simulink model "crazyflie"  (R2019a)
settings: Solver=FixedStepDiscrete  StartTime=0.0  StopTime=25  FixedStep=0.01  RelTol=1e-3
values from neighbouring files (symbols this model uses):
  g = 9.81    [linearization.m]    (also in main.m)
  H = zeros(3,length(idx));  H(1,1) = 1; H(2,2) = 1; H(3,5) = 1    [main.m]
  K_fb_int = K    [main.m]
  K_fb_ref = K    [main.m]
  Kr = pinv( H * inv(eye(size(Ar)) + Br*K_fb_ref - Ar) * Br )    [main.m]
  x0 = [0 0 0  0 0 0  deg2rad(20) deg2rad(20) deg2rad(0) 0 0 0]'    [main.m]
undefined symbols (not defined in the file or in its folder): DiscIntNeverNeededParam
libraries: simulink x2, simulink_extras x1
settings Model: PauseTimes=7  Creator=Zrean  LastModifiedBy=lucas
settings DataIOCC: ReturnWorkspaceOutputs=off
settings OptimizationCC: DefaultParameterBehavior=Inlined  UseDivisionForNetSlopeComputation=on  UseFloatMulNetSlope=on  UseSpecifiedMinMax=on  InlineInvariantSignals=on  PassReuseOutputArgsAs=Individual arguments  ZeroExternalMemoryAtStartup=off  ZeroInternalMemoryAtStartup=off  NoFixptDivByZeroProtection=on  EfficientFloat2IntCast=on  LifeSpan=1
settings DebuggingCC: AlgebraicLoopMsg=error  ParameterTunabilityLossMsg=error  ArithmeticOperatorsInVariantConditions=warning
settings HardwareCC: ProdBitPerPointer=32  ProdBitPerSizeT=32  ProdBitPerPtrDiffT=32  ProdLargestAtomicInteger=Long  ProdLargestAtomicFloat=Double  ProdWordSize=32  ProdHWDeviceType=ARM Compatible->ARM Cortex
settings SFSimCC: SimUseLocalCustomCode=off  MATLABDynamicMemAlloc=off
settings RTWCC: SystemTargetFile=ert.tlc  GenCodeOnly=on  TemplateMakefile=ert_default_tmf  GenerateReport=on  RTWUseLocalCustomCode=off  BuildConfiguration=Faster Runs  IncludeHyperlinkInReport=on  LaunchReport=on  GenerateTraceInfo=on  GenerateTraceReport=on  GenerateTraceReportSl=on  GenerateTraceReportSf=on  GenerateTraceReportEml=on  GenerateCodeMetricsReport=on
settings CodeAppCC: ForceParamTrailComments=on  IgnoreCustomStorageClasses=off  OperatorAnnotations=on  SimulinkDataObjDesc=on  SFDataObjDesc=on  MATLABFcnDesc=on  CustomSymbolStrGlobalVar=rt$N$M  CustomSymbolStrType=$N$M  CustomSymbolStrFcn=$N$M$F  CustomSymbolStrMacro=$N$M  InsertBlockDesc=on  StateflowObjectComments=on  MATLABSourceComments=on
settings ERTTargetCC: TargetLangStandard=C99 (ISO)  MultiwordLength=2048  CombineSignalStateStructs=on  SuppressErrorStatus=on  SupportNonFinite=off  SupportComplex=off  InlinedParameterPlacement=NonHierarchical  ERTCustomFileTemplate=crazyflie_wrapper.tlc  ERTFilePackagingFormat=CompactWithDataFile
settings SimscapeCC: SimscapeNormalizeSystem=off

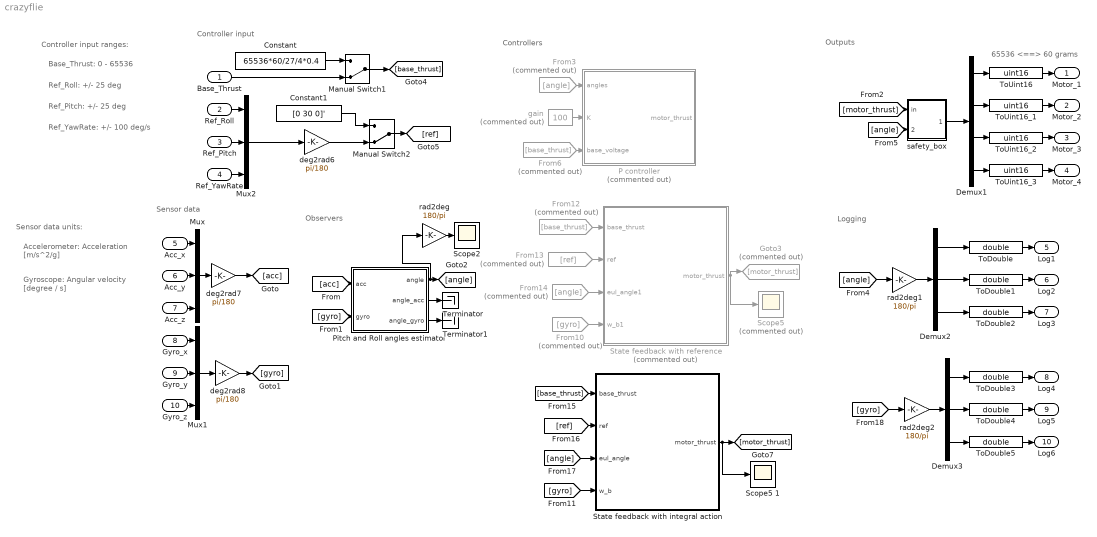
== system crazyflie ==
  note: 65536 <==> 60 grams
  note: Ref_Roll: +/- 25 deg
  note: Base_Thrust: 0 - 65536
  note: Ref_Pitch: +/- 25 deg
  note: Ref_YawRate: +/- 100 deg/s
  note: Controller input ranges:
  note: Gyroscope:
      | Angular velocity [degree / s]
  note: Accelerometer:
      | Acceleration [m/s^2/g]
  note: Sensor data units:
  note: Logging
  note: Outputs
  note: Sensor data
  note: Controllers
  note: Controller input
  note: Observers
  Base_Thrust : Inport  OutDataTypeStr=double
  Ref_Roll : Inport  Port=2  OutDataTypeStr=double
  Ref_Pitch : Inport  Port=3  OutDataTypeStr=double
  Ref_YawRate : Inport  Port=4  OutDataTypeStr=double
  Acc_x : Inport  Port=5  OutDataTypeStr=double  PortDimensions=1
  Acc_y : Inport  Port=6  OutDataTypeStr=double  PortDimensions=1
  Acc_z : Inport  Port=7  OutDataTypeStr=double  PortDimensions=1
  Gyro_x : Inport  Port=8  OutDataTypeStr=double  PortDimensions=1
  Gyro_y : Inport  Port=9  OutDataTypeStr=double  PortDimensions=1
  Gyro_z : Inport  Port=10  OutDataTypeStr=double  PortDimensions=1
  Constant : Constant  Value=65536*60/27/4*0.4
  Constant1 : Constant  Value=[0 30 0]'
  Demux1 : Demux
  Demux2 : Demux  Outputs=3
  Demux3 : Demux  Outputs=3
  From10 : From  Commented=on  GotoTag=gyro
  From12 : From  Commented=on  GotoTag=base_thrust
  From13 : From  Commented=on  GotoTag=ref
  From14 : From  Commented=on  GotoTag=angle
  From3 : From  Commented=on  GotoTag=angle
  From6 : From  Commented=on  GotoTag=base_thrust
  Goto3 : Goto  Commented=on  GotoTag=motor_thrust
  Manual Switch1 : ManualSwitch  CurrentSetting=0
  Manual Switch2 : ManualSwitch  CurrentSetting=0
  Mux : Mux  Inputs=3
  Mux1 : Mux  Inputs=3
  Mux2 : Mux  Inputs=3
  P controller : MATLAB Function  Commented=on  TreatAsAtomicUnit=on
  Pitch and Roll angles estimator : Subsystem
  Scope2 : Scope
  "Scope5 " : Scope  Commented=on
  Scope5 1 : Scope
  State feedback with integral action : Subsystem
  State feedback with reference : Subsystem  Commented=on
  Terminator : Terminator
  Terminator1 : Terminator
  ToDouble{,1..5} (6 alike) : DataTypeConversion  OutDataTypeStr=double  SaturateOnIntegerOverflow=on
  ToUint16 : DataTypeConversion  OutDataTypeStr=uint16  SaturateOnIntegerOverflow=on
  ToUint16_1 : DataTypeConversion  OutDataTypeStr=uint16  SaturateOnIntegerOverflow=on
  ToUint16_2 : DataTypeConversion  OutDataTypeStr=uint16  SaturateOnIntegerOverflow=on
  ToUint16_3 : DataTypeConversion  OutDataTypeStr=uint16  SaturateOnIntegerOverflow=on
  deg2rad6 : Gain  Gain=pi/180
  deg2rad7 : Gain  Gain=pi/180
  deg2rad8 : Gain  Gain=pi/180
  gain : Constant  Commented=on  Value=100
  rad2deg : Gain  Gain=180/pi
  rad2deg1 : Gain  Gain=180/pi
  rad2deg2 : Gain  Gain=180/pi
  safety_box : Subsystem
  Motor_1 : Outport  OutDataTypeStr=uint16  LockScale=on
  Motor_2 : Outport  Port=2  OutDataTypeStr=uint16  LockScale=on
  Motor_3 : Outport  Port=3  OutDataTypeStr=uint16  LockScale=on
  Motor_4 : Outport  Port=4  OutDataTypeStr=uint16  LockScale=on
  Log1 : Outport  Port=5  OutDataTypeStr=double
  Log2 : Outport  Port=6  OutDataTypeStr=double
  Log3 : Outport  Port=7  OutDataTypeStr=double
  Log4 : Outport  Port=8  OutDataTypeStr=double
  Log5 : Outport  Port=9  OutDataTypeStr=double
  Log6 : Outport  Port=10  OutDataTypeStr=double
  wires:
  ToUint16/1 -> Motor_1/1
  ToUint16_1/1 -> Motor_2/1
  ToUint16_2/1 -> Motor_3/1
  ToUint16_3/1 -> Motor_4/1
  ToDouble/1 -> Log1/1
  ToDouble1/1 -> Log2/1
  ToDouble2/1 -> Log3/1
  ToDouble3/1 -> Log4/1
  ToDouble4/1 -> Log5/1
  ToDouble5/1 -> Log6/1
  State feedback with reference/1(motor_thrust) -> Goto3/1, "Scope5 "/1
  [ref] -> State feedback with integral action/2(ref)
  Demux2/3 -> ToDouble2/1
  From12/1 -> State feedback with reference/1(base_thrust)
  [acc] -> Pitch and Roll angles estimator/1(acc)
  State feedback with integral action/1(motor_thrust) -> Scope5 1/1, [motor_thrust]
  Pitch and Roll angles estimator/2(angle_acc) -> Terminator/1
  From6/1 -> P controller/3(base_voltage)
  Pitch and Roll angles estimator/3(angle_gyro) -> Terminator1/1
  Demux2/2 -> ToDouble1/1
  [gyro] -> State feedback with integral action/4(w_b)
  [angle] -> rad2deg1/1
  From3/1 -> P controller/1(angles)
  gain/1 -> P controller/2(K)
  [angle] -> State feedback with integral action/3(eul_angle)
  Pitch and Roll angles estimator/1(angle) -> rad2deg/1, [angle]
  Demux2/1 -> ToDouble/1
  [gyro] -> Pitch and Roll angles estimator/2(gyro)
  [base_thrust] -> State feedback with integral action/1(base_thrust)
  From14/1 -> State feedback with reference/3(eul_angle1)
  From10/1 -> State feedback with reference/4(w_b1)
  From13/1 -> State feedback with reference/2(ref)
  Mux/1 -> deg2rad7/1
  Gyro_z/1 -> Mux1/3
  Acc_x/1 -> Mux/1
  Acc_y/1 -> Mux/2
  Acc_z/1 -> Mux/3
  Gyro_x/1 -> Mux1/1
  Gyro_y/1 -> Mux1/2
  Ref_YawRate/1 -> Mux2/3
  Ref_Pitch/1 -> Mux2/2
  Ref_Roll/1 -> Mux2/1
  Demux1/4 -> ToUint16_3/1
  Demux1/3 -> ToUint16_2/1
  Demux1/2 -> ToUint16_1/1
  Demux1/1 -> ToUint16/1
  Demux3/1 -> ToDouble3/1
  Constant/1 -> Manual Switch1/1
  Mux2/1 -> deg2rad6/1
  Base_Thrust/1 -> Manual Switch1/2
  Manual Switch1/1 -> [base_thrust]
  safety_box/1(Out1) -> Demux1/1
  [angle] -> safety_box/2(angles)
  [motor_thrust] -> safety_box/1(in)
  deg2rad6/1 -> Manual Switch2/2
  deg2rad7/1 -> [acc]
  Mux1/1 -> deg2rad8/1
  deg2rad8/1 -> [gyro]
  rad2deg/1 -> Scope2/1
  [gyro] -> rad2deg2/1
  Demux3/2 -> ToDouble4/1
  Demux3/3 -> ToDouble5/1
  rad2deg1/1 -> Demux2/1
  rad2deg2/1 -> Demux3/1
  Constant1/1 -> Manual Switch2/1
  Manual Switch2/1 -> [ref]

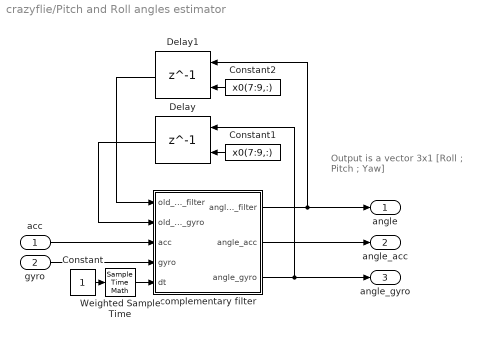
== system crazyflie/Pitch and Roll angles estimator ==
  note: Output is a vector 3x1
      | [Roll ; Pitch ; Yaw]
  acc : Inport
  gyro : Inport  Port=2
  Constant : Constant
  Constant1 : Constant  Value=x0(7:9,:)
  Constant2 : Constant  Value=x0(7:9,:)
  Delay : Delay  DelayLength=1  InitialConditionSource=Input port  InitialCondition=rad2deg(x0(7:9,:))
      settings: InputPortMap=u0,p4
  Delay1 : Delay  DelayLength=1  InitialConditionSource=Input port  InitialCondition=rad2deg(x0(7:9,:))
      settings: InputPortMap=u0,p4
  Weighted Sample Time : SampleTimeMath  TsampMathOp=Ts Only
  complementary filter : MATLAB Function  TreatAsAtomicUnit=on
  angle : Outport
  angle_acc : Outport  Port=2
  angle_gyro : Outport  Port=3
  wires:
  Weighted Sample Time/1 -> complementary filter/5(dt)
  Delay/1 -> complementary filter/2(old_angle_gyro)
  Constant/1 -> Weighted Sample Time/1
  gyro/1 -> complementary filter/4(gyro)
  complementary filter/2(angle_acc) -> angle_acc/1
  complementary filter/3(angle_gyro) -> Delay/1, angle_gyro/1
  acc/1 -> complementary filter/3(acc)
  Constant1/1 -> Delay/2
  Constant2/1 -> Delay1/2
  complementary filter/1(angle_filter) -> Delay1/1, angle/1
  Delay1/1 -> complementary filter/1(old_angle_filter)

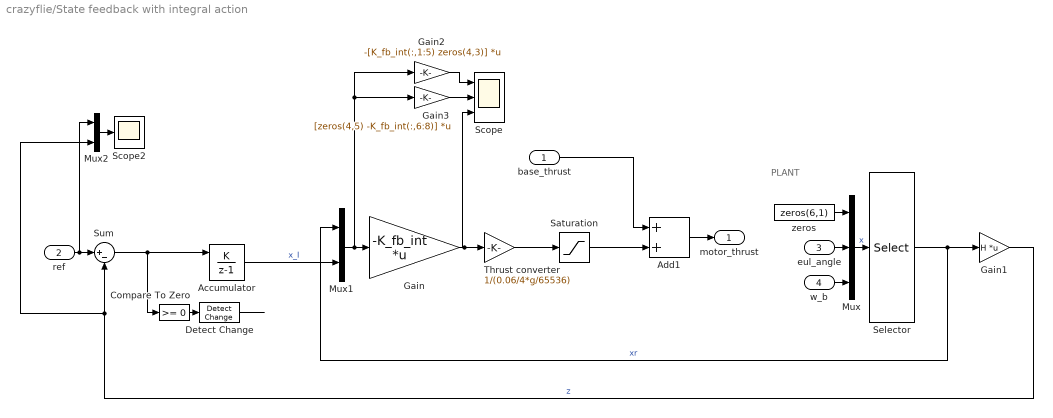
== system crazyflie/State feedback with integral action ==
  note: PLANT
  base_thrust : Inport
  ref : Inport  Port=2
  eul_angle : Inport  Port=3
  w_b : Inport  Port=4
  Accumulator : DiscreteIntegrator  IntegratorMethod=Accumulation: Forward Euler  ExternalReset=either  SampleTime=-1  ICPrevOutput=DiscIntNeverNeededParam  ICPrevScaledInput=DiscIntNeverNeededParam
  Add1 : Sum
  Compare To Zero : simulink/Logic and Bit Operations/Compare To Zero  relop=>=  OutDataTypeStr=boolean
  Detect Change : simulink/Logic and Bit Operations/Detect Change  vinit=0  OutDataTypeStr=boolean
  Gain : Gain  Gain=-K_fb_int  Multiplication=Matrix(K*u)
  Gain1 : Gain  Gain=H  Multiplication=Matrix(K*u)
  Gain2 : Gain  Gain=-[K_fb_int(:,1:5) zeros(4,3)]  Multiplication=Matrix(K*u)
  Gain3 : Gain  Gain=[zeros(4,5) -K_fb_int(:,6:8)]  Multiplication=Matrix(K*u)
  Mux : Mux  Inputs=3
  Mux1 : Mux  Inputs=2
  Mux2 : Mux  Inputs=2
  Saturation : Saturate  UpperLimit=Inf  LowerLimit=0
  Scope : Scope  NumInputPorts=3
  Scope2 : Scope
  Selector : Selector  InputPortWidth=12  IndexOptions=Index vector (dialog)  Indices=idx  OutputSizes=1
  Sum : Sum  Inputs=|+-
  Thrust converter : Gain  Gain=1/(0.06/4*g/65536)
  zeros : Constant  Value=zeros(6,1)
  motor_thrust : Outport
  wires:
  Add1/1 -> motor_thrust/1
  ref/1 -> Mux2/1, Sum/1
  Thrust converter/1 -> Saturation/1
  Mux/1 -> Selector/1  "x"
  Sum/1 -> Compare To Zero/1, Accumulator/1
  Accumulator/1 -> Mux1/2  "x_I"
  Mux1/1 -> Gain2/1, Gain3/1, Gain/1
  Gain/1 -> Scope/3, Thrust converter/1
  eul_angle/1 -> Mux/2
  w_b/1 -> Mux/3
  zeros/1 -> Mux/1
  Gain1/1 -> Mux2/2, Sum/2  "z"
  Selector/1 -> Mux1/1, Gain1/1  "xr"
  base_thrust/1 -> Add1/1
  Compare To Zero/1 -> Detect Change/1
  Detect Change/1 -> ?
  Saturation/1 -> Add1/2
  Gain2/1 -> Scope/1
  Gain3/1 -> Scope/2
  Mux2/1 -> Scope2/1

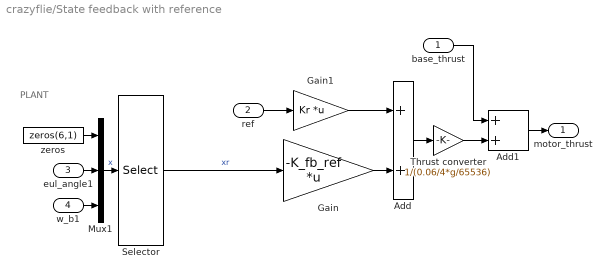
== system crazyflie/State feedback with reference ==
  note: PLANT
  base_thrust : Inport
  ref : Inport  Port=2
  eul_angle1 : Inport  Port=3
  w_b1 : Inport  Port=4
  Add : Sum
  Add1 : Sum
  Gain : Gain  Gain=-K_fb_ref  Multiplication=Matrix(K*u)
  Gain1 : Gain  Gain=Kr  Multiplication=Matrix(K*u)
  Mux1 : Mux  Inputs=3
  Selector : Selector  InputPortWidth=12  IndexOptions=Index vector (dialog)  Indices=idx  OutputSizes=1
  Thrust converter : Gain  Gain=1/(0.06/4*g/65536)
  zeros : Constant  Value=zeros(6,1)
  motor_thrust : Outport
  wires:
  base_thrust/1 -> Add1/1
  Add1/1 -> motor_thrust/1
  ref/1 -> Gain1/1
  Gain1/1 -> Add/1
  Gain/1 -> Add/2
  Add/1 -> Thrust converter/1
  Thrust converter/1 -> Add1/2
  w_b1/1 -> Mux1/3
  zeros/1 -> Mux1/1
  Mux1/1 -> Selector/1  "x"
  eul_angle1/1 -> Mux1/2
  Selector/1 -> Gain/1  "xr"

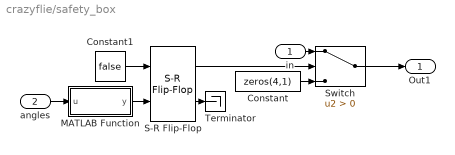
== system crazyflie/safety_box ==
  in : Inport
  angles : Inport  Port=2
  Constant : Constant  Value=zeros(4,1)
  Constant1 : Constant  Value=false
  MATLAB Function : MATLAB Function  TreatAsAtomicUnit=on
  S-R Flip-Flop : simulink_extras/Flip Flops/S-R Flip-Flop  initial_condition=1
  Switch : Switch  Criteria=u2 > Threshold
  Terminator : Terminator
  Out1 : Outport
  wires:
  in/1 -> Switch/1
  Switch/1 -> Out1/1
  Constant/1 -> Switch/3
  angles/1 -> MATLAB Function/1(u)
  MATLAB Function/1(y) -> S-R Flip-Flop/2
  Constant1/1 -> S-R Flip-Flop/1
  S-R Flip-Flop/1 -> Switch/2
  S-R Flip-Flop/2 -> Terminator/1

== matlab function crazyflie/P controller ==
  data: angles input; motor_thrust output; K input; base_voltage input
function motor_thrust  = P_controller(angles, K, base_voltage)

    % initiliaze output
    motor_thrust = zeros(4,1);

    roll_thrust  = K*angles(1);
    pitch_thrust = K*angles(2);
    
    motor_thrust(1) =   roll_thrust + pitch_thrust ;
    motor_thrust(2) =   roll_thrust - pitch_thrust ;
    motor_thrust(3) = - roll_thrust - pitch_thrust ;
    motor_thrust(4) = - roll_thrust + pitch_thrust ;

    motor_thrust = motor_thrust + base_voltage;
    
    motor_thrust = min(65536, max(motor_thrust,0));
  
end

== matlab function crazyflie/Pitch and Roll angles estimator/complementary filter ==
  data: old_angle_filter input; old_angle_gyro input; acc input; angle_filter output; gyro input; dt input; angle_acc output; angle_gyro output
function [angle_filter, angle_acc, angle_gyro] = comp_filter(old_angle_filter, old_angle_gyro, acc, gyro, dt)

    % initialize output
    angle_filter = zeros(3,1);

    %%  tunning parameters
    
    alpha = 0.05;
    gamma = alpha / ( dt + alpha );
%     gamma = 0;
    
    %% Acceleration observer
    
    % normalize acceleration measurements
    if norm(acc) ~= 0
        acc = acc / norm(acc);
    end
    
    % calculate rotation angles based on acceleration sensor
    phi   = atan2(acc(2), acc(3));
    theta = atan2(-acc(1), norm([acc(2), acc(3)] ));
    angle_acc = [phi theta 0]';
    
    
    %% Gyro observer
    
    phi   = old_angle_filter(1);
    theta = old_angle_filter(2);
    psi   = old_angle_filter(3);
    
    rotx  = [1 0        0; 
             0 cos(phi) -sin(phi);
             0 sin(phi) cos(phi)];
    roty  = [cos(theta)  0 sin(theta); 
             0           1 0; 
             -sin(theta) 0 cos(theta)];
    rotz  = [cos(psi) -sin(psi) 0; 
             sin(psi)  cos(psi) 0; 
             0         0        1];
    R_b2w = (rotx * roty * rotz);
    
    T_angleder2w = [ 1,        0,            sin(theta)
                     0, cos(phi),  -cos(theta)*sin(phi)
                     0, sin(phi),   cos(phi)*cos(theta)];
    
    % calculate rotation angles based on gyro sensor
    angle_gyro = old_angle_gyro + dt * inv(T_angleder2w) * R_b2w * gyro; % 
    
    
    %% Sensor Fusion
    
    % fuse acc and gyro sensor to estimate rotation
    angle_filter = (1 - gamma) * angle_acc  + gamma * angle_gyro;

== matlab function crazyflie/safety_box/MATLAB Function ==
  data: u input; y output
function y = fcn(u)

y = abs(u(1)) > deg2rad(60) || abs(u(2)) > deg2rad(60);
